simulink model "bh_4dof_LAGR_manipulator_CONTROL_DL_discrete"  (R2016b)
settings: Solver=ode23s  StartTime=0.0  StopTime=60  FixedStep=0.001  RelTol=1e-5  EnableMultiTasking=on
StopFcn:
  | bh_4dof_sim_post_process
values from neighbouring files (symbols this model uses):
  N = 3    [bh_4dof_sim_post_process.m]
undefined symbols (not defined in the file or in its folder): b1_damp, b2_damp, b3_damp, b4_damp, g, Hz, L1x, L1y, L1z, L2x, L2y, L2z, L3x, L3y, L3z, mass1, mass2, mass3, mass4, Rturn, theta1_0, theta1_dot_0, theta2_0, theta2_dot_0, theta3_0, theta3_dot_0, theta4_0, theta4_dot_0, X, Y, Z
libraries: simulink_extras x42, sm_lib x25, simulink x18, nesl_utility x17, discretizing x8
(part 4 of 4)

== system bh_4dof_LAGR_manipulator_CONTROL_DL_discrete/SIMULINK_MODEL/inside_MCKGQ/Subsystem1 ==
  M : Inport
  C : Inport  Port=2
  K : Inport  Port=3
  G : Inport  Port=4
  Q : Inport  Port=5
  T : Inport  Port=6
  Bus Selector : BusSelector  OutputSignals=theta_DOT_col
  Bus Selector1 : BusSelector  OutputSignals=theta_col
  Demux : Demux
  MATLAB Function : MATLAB Function  TreatAsAtomicUnit=on
  Product : Product  Multiplication=Matrix(*)
  Product1 : Product  Multiplication=Matrix(*)
  Product2 : Product  Inputs=/  Multiplication=Matrix(*)
  Product3 : Product  Multiplication=Matrix(*)
  SC_cond : Scope
  Sum : Sum  Inputs=+|+|+
  Sum1 : Sum  Inputs=|-+
  TH1_DD : Outport
  TH2_DD : Outport  Port=2
  TH3_DD : Outport  Port=3
  TH4_DD : Outport  Port=4
  wires:
  T/1 -> [T]
  C/1 -> Product/1
  [T] -> Bus Selector/1
  Bus Selector/1 -> Product/2  "<theta_DOT_col>"
  K/1 -> Product1/1
  [T] -> Bus Selector1/1
  Bus Selector1/1 -> Product1/2  "<theta_col>"
  Q/1 -> Sum1/2
  Product1/1 -> Sum/2
  G/1 -> Sum/3
  Product/1 -> Sum/1
  Sum/1 -> Sum1/1
  M/1 -> Product2/1, MATLAB Function/1(M)
  Product2/1 -> Product3/1
  Sum1/1 -> Product3/2
  Product3/1 -> Demux/1
  Demux/1 -> TH1_DD/1
  Demux/2 -> TH2_DD/1
  MATLAB Function/1(the_cond) -> SC_cond/1
  Demux/3 -> TH3_DD/1
  Demux/4 -> TH4_DD/1

== matlab function bh_4dof_LAGR_manipulator_CONTROL_DL_discrete/TRAJECTORY/THE_J ==
  data: L1Y_s input; the_J output; L2Y_s input; L3Y_s input; theta1 input; theta2 input; theta3 input; theta4 input
function the_J = THE_J(L1Y_s,L2Y_s,L3Y_s,theta1,theta2,theta3,theta4)
%#codegen

%    This function was generated by the Symbolic Math Toolbox version 7.0.
%    13-Sep-2016 14:49:06

the_J = reshape([sin(theta4).*(L2Y_s.*sin(theta1+theta2)+L1Y_s.*sin(theta1)+L3Y_s.*sin(theta1+theta2+theta3)),-cos(theta4).*(L2Y_s.*sin(theta1+theta2)+L1Y_s.*sin(theta1)+L3Y_s.*sin(theta1+theta2+theta3)),L2Y_s.*cos(theta1+theta2)+L1Y_s.*cos(theta1)+L3Y_s.*cos(theta1+theta2+theta3),sin(theta4).*(L2Y_s.*sin(theta1+theta2)+L3Y_s.*sin(theta1+theta2+theta3)),-cos(theta4).*(L2Y_s.*sin(theta1+theta2)+L3Y_s.*sin(theta1+theta2+theta3)),L2Y_s.*cos(theta1+theta2)+L3Y_s.*cos(theta1+theta2+theta3),L3Y_s.*sin(theta1+theta2+theta3).*sin(theta4),-L3Y_s.*sin(theta1+theta2+theta3).*cos(theta4),L3Y_s.*cos(theta1+theta2+theta3),-cos(theta4).*(L2Y_s.*cos(theta1+theta2)+L1Y_s.*cos(theta1)+L3Y_s.*cos(theta1+theta2+theta3)),-sin(theta4).*(L2Y_s.*cos(theta1+theta2)+L1Y_s.*cos(theta1)+L3Y_s.*cos(theta1+theta2+theta3)),0.0],[3,4]);

== matlab function bh_4dof_LAGR_manipulator_CONTROL_DL_discrete/Create_PLANT_BUS1/CALC_BUS/THE_A_EFF_and_O_and_G ==
  data: L1Y_s input; AF_pos_eff output; L2Y_s input; L3Y_s input; theta1 input; theta2 input; theta3 input; AF_pos_O1 output; AF_pos_O2 output; AF_pos_O3 output; AF_pos_G1 output; AF_pos_G2 output; AF_pos_G3 output
function [AF_pos_eff,AF_pos_O1,AF_pos_O2,AF_pos_O3,AF_pos_G1,AF_pos_G2,AF_pos_G3] = THE_A_EFF_and_O_and_G(L1Y_s,L2Y_s,L3Y_s,theta1,theta2,theta3)
%#codegen

%    This function was generated by the Symbolic Math Toolbox version 7.0.
%    15-Sep-2016 15:54:05

AF_pos_eff = [0.0;L2Y_s.*cos(theta1+theta2)+L1Y_s.*cos(theta1)+L3Y_s.*cos(theta1+theta2+theta3);L2Y_s.*sin(theta1+theta2)+L1Y_s.*sin(theta1)+L3Y_s.*sin(theta1+theta2+theta3)];
if nargout > 1
    AF_pos_O1 = [0.0;0.0;0.0];
end
if nargout > 2
    AF_pos_O2 = [0.0;L1Y_s.*cos(theta1);L1Y_s.*sin(theta1)];
end
if nargout > 3
    AF_pos_O3 = [0.0;L2Y_s.*cos(theta1+theta2)+L1Y_s.*cos(theta1);L2Y_s.*sin(theta1+theta2)+L1Y_s.*sin(theta1)];
end
if nargout > 4
    AF_pos_G1 = [0.0;L1Y_s.*cos(theta1).*(1.0./2.0);L1Y_s.*sin(theta1).*(1.0./2.0)];
end
if nargout > 5
    AF_pos_G2 = [0.0;L2Y_s.*cos(theta1+theta2).*(1.0./2.0)+L1Y_s.*cos(theta1);L2Y_s.*sin(theta1+theta2).*(1.0./2.0)+L1Y_s.*sin(theta1)];
end
if nargout > 6
    AF_pos_G3 = [0.0;L2Y_s.*cos(theta1+theta2)+L1Y_s.*cos(theta1)+L3Y_s.*cos(theta1+theta2+theta3).*(1.0./2.0);L2Y_s.*sin(theta1+theta2)+L1Y_s.*sin(theta1)+L3Y_s.*sin(theta1+theta2+theta3).*(1.0./2.0)];
end

== matlab function bh_4dof_LAGR_manipulator_CONTROL_DL_discrete/TRAJECTORY/CALC_THETA_DOT ==
  data: J input; TH_DOT output; XY_DOT input; lambda_sq input; alt_TH_DOT output
function [TH_DOT, alt_TH_DOT] = calc_TH_DOT(J, XY_DOT, lambda_sq)
%#codegen

    %% so our problem is this:
    %     J*q_dot = x_dot
    %
    % so a solution is:
    %
    %      q_dot = pinv(J) * x_dot
    
    TH_DOT = pinv(J) * XY_DOT;

    %% we can also penalise the q_dot by applying a weight to it.
    %  this will give us a solution where we get a "smaller" q_dot.  This
    %  acts as a "dampening" agent ... and we notice it most at startup.
    
    % consider solving the REGULARISED problem
    %     [       J_mxn  ] * q_dot =  [ x_dot ]
    %     [lamb^2*I_nxn  ]            [ 0_nx1 ]
    %
    % which we'll wite as:
    %
    %              new_A * q_dot = new_b
    %
    % so a solution is:
    %
    %      q_dot = pinv(new_A) * new_b
    
    [m, n]     = size(J); 
    I_mat      = eye( n ); 
    new_A      = [ J;
                   lambda_sq * I_mat];

    new_b      = [ XY_DOT;
                   zeros(n,1) ];

    alt_TH_DOT = pinv( new_A  ) * new_b;
end

== matlab function bh_4dof_LAGR_manipulator_CONTROL_DL_discrete/SIMULINK_MODEL/inside_MCKGQ/Subsystem1/MATLAB Function ==
  data: M input; the_cond output
function the_cond = COND(M)
%#codegen

the_cond = cond(M);

end

== matlab function bh_4dof_LAGR_manipulator_CONTROL_DL_discrete/Create_PLANT_BUS1/CALC_BUS/THE_W_EFF_and_O_and_G ==
  data: L1Y_s input; WF_pos_eff output; L2Y_s input; L3Y_s input; theta1 input; theta2 input; theta3 input; theta4 input; WF_pos_O1 output; WF_pos_O2 output; WF_pos_O3 output; WF_pos_G1 output; WF_pos_G2 output; WF_pos_G3 output
function [WF_pos_eff,WF_pos_O1,WF_pos_O2,WF_pos_O3,WF_pos_G1,WF_pos_G2,WF_pos_G3] = THE_W_EFF_and_O_and_G(L1Y_s,L2Y_s,L3Y_s,theta1,theta2,theta3,theta4)
%#codegen

%    This function was generated by the Symbolic Math Toolbox version 7.0.
%    15-Sep-2016 15:32:27

WF_pos_eff = [-sin(theta4).*(L2Y_s.*cos(theta1+theta2)+L1Y_s.*cos(theta1)+L3Y_s.*cos(theta1+theta2+theta3));cos(theta4).*(L2Y_s.*cos(theta1+theta2)+L1Y_s.*cos(theta1)+L3Y_s.*cos(theta1+theta2+theta3));L2Y_s.*sin(theta1+theta2)+L1Y_s.*sin(theta1)+L3Y_s.*sin(theta1+theta2+theta3)];
if nargout > 1
    WF_pos_O1 = [0.0;0.0;0.0];
end
if nargout > 2
    WF_pos_O2 = [-L1Y_s.*cos(theta1).*sin(theta4);L1Y_s.*cos(theta1).*cos(theta4);L1Y_s.*sin(theta1)];
end
if nargout > 3
    WF_pos_O3 = [-sin(theta4).*(L2Y_s.*cos(theta1+theta2)+L1Y_s.*cos(theta1));cos(theta4).*(L2Y_s.*cos(theta1+theta2)+L1Y_s.*cos(theta1));L2Y_s.*sin(theta1+theta2)+L1Y_s.*sin(theta1)];
end
if nargout > 4
    WF_pos_G1 = [L1Y_s.*cos(theta1).*sin(theta4).*(-1.0./2.0);L1Y_s.*cos(theta1).*cos(theta4).*(1.0./2.0);L1Y_s.*sin(theta1).*(1.0./2.0)];
end
if nargout > 5
    WF_pos_G2 = [-sin(theta4).*(L2Y_s.*cos(theta1+theta2).*(1.0./2.0)+L1Y_s.*cos(theta1));cos(theta4).*(L2Y_s.*cos(theta1+theta2).*(1.0./2.0)+L1Y_s.*cos(theta1));L2Y_s.*sin(theta1+theta2).*(1.0./2.0)+L1Y_s.*sin(theta1)];
end
if nargout > 6
    WF_pos_G3 = [-sin(theta4).*(L2Y_s.*cos(theta1+theta2)+L1Y_s.*cos(theta1)+L3Y_s.*cos(theta1+theta2+theta3).*(1.0./2.0));cos(theta4).*(L2Y_s.*cos(theta1+theta2)+L1Y_s.*cos(theta1)+L3Y_s.*cos(theta1+theta2+theta3).*(1.0./2.0));L2Y_s.*sin(theta1+theta2)+L1Y_s.*sin(theta1)+L3Y_s.*sin(theta1+theta2+theta3).*(1.0./2.0)];
end

== matlab function bh_4dof_LAGR_manipulator_CONTROL_DL_discrete/Create_PLANT_BUS1/Subsystem1/MATLAB Function ==
  data: r input size=[3 1]; TQ output; F input size=[3 1]
function TQ = CROSS(r,F)
%#codegen

TQ = cross(r,F);

== matlab function bh_4dof_LAGR_manipulator_CONTROL_DL_discrete/Create_PLANT_BUS1/Subsystem1/MATLAB Function1 ==
  data: r input size=[3 1]; TQ output; F input size=[3 1]
function TQ = CROSS(r,F)
%#codegen

TQ = cross(r,F);

== matlab function bh_4dof_LAGR_manipulator_CONTROL_DL_discrete/Create_PLANT_BUS1/Subsystem1/MATLAB Function2 ==
  data: r input size=[3 1]; TQ output; F input size=[3 1]
function TQ = CROSS(r,F)
%#codegen

TQ = cross(r,F);

== matlab function bh_4dof_LAGR_manipulator_CONTROL_DL_discrete/Create_PLANT_BUS1/Subsystem1/MATLAB Function3 ==
  data: r input size=[3 1]; TQ output; F input size=[3 1]
function TQ = CROSS(r,F)
%#codegen

TQ = cross(r,F);

== matlab function bh_4dof_LAGR_manipulator_CONTROL_DL_discrete/Create_PLANT_BUS1/Subsystem1/MATLAB Function4 ==
  data: r input size=[3 1]; TQ output; F input size=[3 1]
function TQ = CROSS(r,F)
%#codegen

TQ = cross(r,F);

== matlab function bh_4dof_LAGR_manipulator_CONTROL_DL_discrete/Create_PLANT_BUS1/Subsystem1/MATLAB Function5 ==
  data: r input size=[3 1]; TQ output; F input size=[3 1]
function TQ = CROSS(r,F)
%#codegen

TQ = cross(r,F);

== matlab function bh_4dof_LAGR_manipulator_CONTROL_DL_discrete/TRAJECTORY/THE_XEYE ==
  data: L1Y_s input; XE output; L2Y_s input; L3Y_s input; theta1 input; theta2 input; theta3 input; theta4 input; YE output; ZE output
function [XE,YE,ZE] = THE_XEYE(L1Y_s,L2Y_s,L3Y_s,theta1,theta2,theta3,theta4)
%#codegen

%    This function was generated by the Symbolic Math Toolbox version 7.0.
%    13-Sep-2016 15:29:58

XE = -sin(theta4).*(L2Y_s.*cos(theta1+theta2)+L1Y_s.*cos(theta1)+L3Y_s.*cos(theta1+theta2+theta3));
if nargout > 1
    YE = cos(theta4).*(L2Y_s.*cos(theta1+theta2)+L1Y_s.*cos(theta1)+L3Y_s.*cos(theta1+theta2+theta3));
end
if nargout > 2
    ZE = L2Y_s.*sin(theta1+theta2)+L1Y_s.*sin(theta1)+L3Y_s.*sin(theta1+theta2+theta3);
end

== matlab function bh_4dof_LAGR_manipulator_CONTROL_DL_discrete/Create_PLANT_BUS/CALC_BUS/THE_A_EFF_and_O_and_G ==
  data: L1Y_s input; AF_pos_eff output; L2Y_s input; L3Y_s input; theta1 input; theta2 input; theta3 input; AF_pos_O1 output; AF_pos_O2 output; AF_pos_O3 output; AF_pos_G1 output; AF_pos_G2 output; AF_pos_G3 output
function [AF_pos_eff,AF_pos_O1,AF_pos_O2,AF_pos_O3,AF_pos_G1,AF_pos_G2,AF_pos_G3] = THE_A_EFF_and_O_and_G(L1Y_s,L2Y_s,L3Y_s,theta1,theta2,theta3)
%#codegen

%    This function was generated by the Symbolic Math Toolbox version 7.0.
%    15-Sep-2016 15:54:05

AF_pos_eff = [0.0;L2Y_s.*cos(theta1+theta2)+L1Y_s.*cos(theta1)+L3Y_s.*cos(theta1+theta2+theta3);L2Y_s.*sin(theta1+theta2)+L1Y_s.*sin(theta1)+L3Y_s.*sin(theta1+theta2+theta3)];
if nargout > 1
    AF_pos_O1 = [0.0;0.0;0.0];
end
if nargout > 2
    AF_pos_O2 = [0.0;L1Y_s.*cos(theta1);L1Y_s.*sin(theta1)];
end
if nargout > 3
    AF_pos_O3 = [0.0;L2Y_s.*cos(theta1+theta2)+L1Y_s.*cos(theta1);L2Y_s.*sin(theta1+theta2)+L1Y_s.*sin(theta1)];
end
if nargout > 4
    AF_pos_G1 = [0.0;L1Y_s.*cos(theta1).*(1.0./2.0);L1Y_s.*sin(theta1).*(1.0./2.0)];
end
if nargout > 5
    AF_pos_G2 = [0.0;L2Y_s.*cos(theta1+theta2).*(1.0./2.0)+L1Y_s.*cos(theta1);L2Y_s.*sin(theta1+theta2).*(1.0./2.0)+L1Y_s.*sin(theta1)];
end
if nargout > 6
    AF_pos_G3 = [0.0;L2Y_s.*cos(theta1+theta2)+L1Y_s.*cos(theta1)+L3Y_s.*cos(theta1+theta2+theta3).*(1.0./2.0);L2Y_s.*sin(theta1+theta2)+L1Y_s.*sin(theta1)+L3Y_s.*sin(theta1+theta2+theta3).*(1.0./2.0)];
end

== matlab function bh_4dof_LAGR_manipulator_CONTROL_DL_discrete/Create_PLANT_BUS/CALC_BUS/THE_W_EFF_and_O_and_G ==
  data: L1Y_s input; WF_pos_eff output; L2Y_s input; L3Y_s input; theta1 input; theta2 input; theta3 input; theta4 input; WF_pos_O1 output; WF_pos_O2 output; WF_pos_O3 output; WF_pos_G1 output; WF_pos_G2 output; WF_pos_G3 output
function [WF_pos_eff,WF_pos_O1,WF_pos_O2,WF_pos_O3,WF_pos_G1,WF_pos_G2,WF_pos_G3] = THE_W_EFF_and_O_and_G(L1Y_s,L2Y_s,L3Y_s,theta1,theta2,theta3,theta4)
%#codegen

%    This function was generated by the Symbolic Math Toolbox version 7.0.
%    15-Sep-2016 15:32:27

WF_pos_eff = [-sin(theta4).*(L2Y_s.*cos(theta1+theta2)+L1Y_s.*cos(theta1)+L3Y_s.*cos(theta1+theta2+theta3));cos(theta4).*(L2Y_s.*cos(theta1+theta2)+L1Y_s.*cos(theta1)+L3Y_s.*cos(theta1+theta2+theta3));L2Y_s.*sin(theta1+theta2)+L1Y_s.*sin(theta1)+L3Y_s.*sin(theta1+theta2+theta3)];
if nargout > 1
    WF_pos_O1 = [0.0;0.0;0.0];
end
if nargout > 2
    WF_pos_O2 = [-L1Y_s.*cos(theta1).*sin(theta4);L1Y_s.*cos(theta1).*cos(theta4);L1Y_s.*sin(theta1)];
end
if nargout > 3
    WF_pos_O3 = [-sin(theta4).*(L2Y_s.*cos(theta1+theta2)+L1Y_s.*cos(theta1));cos(theta4).*(L2Y_s.*cos(theta1+theta2)+L1Y_s.*cos(theta1));L2Y_s.*sin(theta1+theta2)+L1Y_s.*sin(theta1)];
end
if nargout > 4
    WF_pos_G1 = [L1Y_s.*cos(theta1).*sin(theta4).*(-1.0./2.0);L1Y_s.*cos(theta1).*cos(theta4).*(1.0./2.0);L1Y_s.*sin(theta1).*(1.0./2.0)];
end
if nargout > 5
    WF_pos_G2 = [-sin(theta4).*(L2Y_s.*cos(theta1+theta2).*(1.0./2.0)+L1Y_s.*cos(theta1));cos(theta4).*(L2Y_s.*cos(theta1+theta2).*(1.0./2.0)+L1Y_s.*cos(theta1));L2Y_s.*sin(theta1+theta2).*(1.0./2.0)+L1Y_s.*sin(theta1)];
end
if nargout > 6
    WF_pos_G3 = [-sin(theta4).*(L2Y_s.*cos(theta1+theta2)+L1Y_s.*cos(theta1)+L3Y_s.*cos(theta1+theta2+theta3).*(1.0./2.0));cos(theta4).*(L2Y_s.*cos(theta1+theta2)+L1Y_s.*cos(theta1)+L3Y_s.*cos(theta1+theta2+theta3).*(1.0./2.0));L2Y_s.*sin(theta1+theta2)+L1Y_s.*sin(theta1)+L3Y_s.*sin(theta1+theta2+theta3).*(1.0./2.0)];
end

== matlab function bh_4dof_LAGR_manipulator_CONTROL_DL_discrete/Create_PLANT_BUS/Subsystem1/MATLAB Function ==
  data: r input size=[3 1]; TQ output; F input size=[3 1]
function TQ = CROSS(r,F)
%#codegen

TQ = cross(r,F);

== matlab function bh_4dof_LAGR_manipulator_CONTROL_DL_discrete/Create_PLANT_BUS/Subsystem1/MATLAB Function1 ==
  data: r input size=[3 1]; TQ output; F input size=[3 1]
function TQ = CROSS(r,F)
%#codegen

TQ = cross(r,F);

== matlab function bh_4dof_LAGR_manipulator_CONTROL_DL_discrete/Create_PLANT_BUS/Subsystem1/MATLAB Function2 ==
  data: r input size=[3 1]; TQ output; F input size=[3 1]
function TQ = CROSS(r,F)
%#codegen

TQ = cross(r,F);

== matlab function bh_4dof_LAGR_manipulator_CONTROL_DL_discrete/Create_PLANT_BUS/Subsystem1/MATLAB Function3 ==
  data: r input size=[3 1]; TQ output; F input size=[3 1]
function TQ = CROSS(r,F)
%#codegen

TQ = cross(r,F);

== matlab function bh_4dof_LAGR_manipulator_CONTROL_DL_discrete/Create_PLANT_BUS/Subsystem1/MATLAB Function4 ==
  data: r input size=[3 1]; TQ output; F input size=[3 1]
function TQ = CROSS(r,F)
%#codegen

TQ = cross(r,F);

== matlab function bh_4dof_LAGR_manipulator_CONTROL_DL_discrete/Create_PLANT_BUS/Subsystem1/MATLAB Function5 ==
  data: r input size=[3 1]; TQ output; F input size=[3 1]
function TQ = CROSS(r,F)
%#codegen

TQ = cross(r,F);

== matlab function bh_4dof_LAGR_manipulator_CONTROL_DL_discrete/SIMULINK_MODEL/inside_MCKGQ/MCKGQ ==
  data: L1X_s input; M output; L2X_s input; L3X_s input; L1Y_s input; L2Y_s input; L3Y_s input; L1Z_s input; L2Z_s input; L3Z_s input; R4_s input; TH1_s input; TH2_s input; TH3_s input; TH1_s_D input; TH2_s_D input; TH3_s_D input; TH4_s_D input; b1_s input; b2_s input; b3_s input; b4_s input; g_s input; m1_s input; m2_s input; m3_s input; m4_s input; taum1_s input; taum2_s input; taum3_s input; taum4_s input; C output; K output; G output; Q output
function [M,C,K,G,Q] = MCKGQ(L1X_s,L2X_s,L3X_s,L1Y_s,L2Y_s,L3Y_s,L1Z_s,L2Z_s,L3Z_s,R4_s,TH1_s,TH2_s,TH3_s,TH1_s_D,TH2_s_D,TH3_s_D,TH4_s_D,b1_s,b2_s,b3_s,b4_s,g_s,m1_s,m2_s,m3_s,m4_s,taum1_s,taum2_s,taum3_s,taum4_s)
%#codegen

%    This function was generated by the Symbolic Math Toolbox version 7.1.
%    31-Jan-2017 14:34:44

M = reshape([L1Y_s.^2.*m1_s.*(1.0./3.0)+L1Y_s.^2.*m2_s+L1Y_s.^2.*m3_s+L2Y_s.^2.*m2_s.*(1.0./3.0)+L2Y_s.^2.*m3_s+L3Y_s.^2.*m3_s.*(1.0./3.0)+L1Z_s.^2.*m1_s.*(1.0./1.2e1)+L2Z_s.^2.*m2_s.*(1.0./1.2e1)+L3Z_s.^2.*m3_s.*(1.0./1.2e1)+L1Y_s.*L2Y_s.*m2_s.*cos(TH2_s)+L1Y_s.*L2Y_s.*m3_s.*cos(TH2_s).*2.0+L2Y_s.*L3Y_s.*m3_s.*cos(TH3_s)+L1Y_s.*L3Y_s.*m3_s.*cos(TH2_s+TH3_s),L2Y_s.^2.*m2_s.*(1.0./3.0)+L2Y_s.^2.*m3_s+L3Y_s.^2.*m3_s.*(1.0./3.0)+L2Z_s.^2.*m2_s.*(1.0./1.2e1)+L3Z_s.^2.*m3_s.*(1.0./1.2e1)+L1Y_s.*L2Y_s.*m2_s.*cos(TH2_s).*(1.0./2.0)+L1Y_s.*L2Y_s.*m3_s.*cos(TH2_s)+L2Y_s.*L3Y_s.*m3_s.*cos(TH3_s)+L1Y_s.*L3Y_s.*m3_s.*cos(TH2_s+TH3_s).*(1.0./2.0),m3_s.*(L3Y_s.^2.*4.0+L3Z_s.^2+L1Y_s.*L3Y_s.*cos(TH2_s+TH3_s).*6.0+L2Y_s.*L3Y_s.*cos(TH3_s).*6.0).*(1.0./1.2e1),0.0,L2Y_s.^2.*m2_s.*(1.0./3.0)+L2Y_s.^2.*m3_s+L3Y_s.^2.*m3_s.*(1.0./3.0)+L2Z_s.^2.*m2_s.*(1.0./1.2e1)+L3Z_s.^2.*m3_s.*(1.0./1.2e1)+L1Y_s.*L2Y_s.*m2_s.*cos(TH2_s).*(1.0./2.0)+L1Y_s.*L2Y_s.*m3_s.*cos(TH2_s)+L2Y_s.*L3Y_s.*m3_s.*cos(TH3_s)+L1Y_s.*L3Y_s.*m3_s.*cos(TH2_s+TH3_s).*(1.0./2.0),L2Y_s.^2.*m2_s.*(1.0./3.0)+L2Y_s.^2.*m3_s+L3Y_s.^2.*m3_s.*(1.0./3.0)+L2Z_s.^2.*m2_s.*(1.0./1.2e1)+L3Z_s.^2.*m3_s.*(1.0./1.2e1)+L2Y_s.*L3Y_s.*m3_s.*cos(TH3_s),m3_s.*(L3Y_s.^2.*4.0+L3Z_s.^2+L2Y_s.*L3Y_s.*cos(TH3_s).*6.0).*(1.0./1.2e1),0.0,m3_s.*(L3Y_s.^2.*4.0+L3Z_s.^2+L1Y_s.*L3Y_s.*cos(TH2_s+TH3_s).*6.0+L2Y_s.*L3Y_s.*cos(TH3_s).*6.0).*(1.0./1.2e1),m3_s.*(L3Y_s.^2.*4.0+L3Z_s.^2+L2Y_s.*L3Y_s.*cos(TH3_s).*6.0).*(1.0./1.2e1),m3_s.*(L3Y_s.^2.*4.0+L3Z_s.^2).*(1.0./1.2e1),0.0,0.0,0.0,0.0,L1X_s.^2.*m1_s.*(1.0./1.2e1)+L2X_s.^2.*m2_s.*(1.0./1.2e1)+L3X_s.^2.*m3_s.*(1.0./1.2e1)+L1Y_s.^2.*m1_s.*(1.0./6.0)+L1Y_s.^2.*m2_s.*(1.0./2.0)+L1Y_s.^2.*m3_s.*(1.0./2.0)+L2Y_s.^2.*m2_s.*(1.0./6.0)+L2Y_s.^2.*m3_s.*(1.0./2.0)+L3Y_s.^2.*m3_s.*(1.0./6.0)+L1Z_s.^2.*m1_s.*(1.0./2.4e1)+L2Z_s.^2.*m2_s.*(1.0./2.4e1)+L3Z_s.^2.*m3_s.*(1.0./2.4e1)+R4_s.^2.*m4_s.*(1.0./2.0)+L3Y_s.^2.*m3_s.*cos(TH1_s.*2.0+TH2_s.*2.0+TH3_s.*2.0).*(1.0./6.0)-L3Z_s.^2.*m3_s.*cos(TH1_s.*2.0+TH2_s.*2.0+TH3_s.*2.0).*(1.0./2.4e1)+L1Y_s.^2.*m1_s.*cos(TH1_s.*2.0).*(1.0./6.0)+L1Y_s.^2.*m2_s.*cos(TH1_s.*2.0).*(1.0./2.0)+L1Y_s.^2.*m3_s.*cos(TH1_s.*2.0).*(1.0./2.0)-L1Z_s.^2.*m1_s.*cos(TH1_s.*2.0).*(1.0./2.4e1)+L2Y_s.^2.*m2_s.*cos(TH1_s.*2.0+TH2_s.*2.0).*(1.0./6.0)+L2Y_s.^2.*m3_s.*cos(TH1_s.*2.0+TH2_s.*2.0).*(1.0./2.0)-L2Z_s.^2.*m2_s.*cos(TH1_s.*2.0+TH2_s.*2.0).*(1.0./2.4e1)+L1Y_s.*L2Y_s.*m2_s.*cos(TH2_s).*(1.0./2.0)+L1Y_s.*L2Y_s.*m3_s.*cos(TH2_s)+L2Y_s.*L3Y_s.*m3_s.*cos(TH3_s).*(1.0./2.0)+L1Y_s.*L2Y_s.*m2_s.*cos(TH1_s.*2.0+TH2_s).*(1.0./2.0)+L1Y_s.*L2Y_s.*m3_s.*cos(TH1_s.*2.0+TH2_s)+L1Y_s.*L3Y_s.*m3_s.*cos(TH1_s.*2.0+TH2_s+TH3_s).*(1.0./2.0)+L1Y_s.*L3Y_s.*m3_s.*cos(TH2_s+TH3_s).*(1.0./2.0)+L2Y_s.*L3Y_s.*m3_s.*cos(TH1_s.*2.0+TH2_s.*2.0+TH3_s).*(1.0./2.0)],[4,4]);
if nargout > 1
    C = reshape([-L1Y_s.*L3Y_s.*TH2_s_D.*m3_s.*sin(TH2_s+TH3_s)-L1Y_s.*L3Y_s.*TH3_s_D.*m3_s.*sin(TH2_s+TH3_s)-L1Y_s.*L2Y_s.*TH2_s_D.*m2_s.*sin(TH2_s)-L1Y_s.*L2Y_s.*TH2_s_D.*m3_s.*sin(TH2_s).*2.0-L2Y_s.*L3Y_s.*TH3_s_D.*m3_s.*sin(TH3_s),L1Y_s.*L3Y_s.*TH1_s_D.*m3_s.*sin(TH2_s+TH3_s).*(1.0./2.0)+L1Y_s.*L2Y_s.*TH1_s_D.*m2_s.*sin(TH2_s).*(1.0./2.0)+L1Y_s.*L2Y_s.*TH1_s_D.*m3_s.*sin(TH2_s)-L2Y_s.*L3Y_s.*TH3_s_D.*m3_s.*sin(TH3_s),L3Y_s.*m3_s.*(L1Y_s.*TH1_s_D.*sin(TH2_s+TH3_s)+L2Y_s.*TH1_s_D.*sin(TH3_s)+L2Y_s.*TH2_s_D.*sin(TH3_s).*2.0).*(1.0./2.0),TH4_s_D.*(L3Y_s.^2.*m3_s.*sin(TH1_s.*2.0+TH2_s.*2.0+TH3_s.*2.0).*4.0-L3Z_s.^2.*m3_s.*sin(TH1_s.*2.0+TH2_s.*2.0+TH3_s.*2.0)+L1Y_s.^2.*m1_s.*sin(TH1_s.*2.0).*4.0+L1Y_s.^2.*m2_s.*sin(TH1_s.*2.0).*1.2e1+L1Y_s.^2.*m3_s.*sin(TH1_s.*2.0).*1.2e1-L1Z_s.^2.*m1_s.*sin(TH1_s.*2.0)+L2Y_s.^2.*m2_s.*sin(TH1_s.*2.0+TH2_s.*2.0).*4.0+L2Y_s.^2.*m3_s.*sin(TH1_s.*2.0+TH2_s.*2.0).*1.2e1-L2Z_s.^2.*m2_s.*sin(TH1_s.*2.0+TH2_s.*2.0)+L1Y_s.*L2Y_s.*m2_s.*sin(TH1_s.*2.0+TH2_s).*1.2e1+L1Y_s.*L2Y_s.*m3_s.*sin(TH1_s.*2.0+TH2_s).*2.4e1+L1Y_s.*L3Y_s.*m3_s.*sin(TH1_s.*2.0+TH2_s+TH3_s).*1.2e1+L2Y_s.*L3Y_s.*m3_s.*sin(TH1_s.*2.0+TH2_s.*2.0+TH3_s).*1.2e1).*(-1.0./1.2e1),L1Y_s.*L3Y_s.*TH2_s_D.*m3_s.*sin(TH2_s+TH3_s).*(-1.0./2.0)-L1Y_s.*L3Y_s.*TH3_s_D.*m3_s.*sin(TH2_s+TH3_s)-L1Y_s.*L2Y_s.*TH2_s_D.*m2_s.*sin(TH2_s).*(1.0./2.0)-L1Y_s.*L2Y_s.*TH2_s_D.*m3_s.*sin(TH2_s)-L2Y_s.*L3Y_s.*TH3_s_D.*m3_s.*sin(TH3_s),-L2Y_s.*L3Y_s.*TH3_s_D.*m3_s.*sin(TH3_s),L2Y_s.*L3Y_s.*TH2_s_D.*m3_s.*sin(TH3_s).*(1.0./2.0),TH4_s_D.*(L3Y_s.^2.*m3_s.*sin(TH1_s.*2.0+TH2_s.*2.0+TH3_s.*2.0).*4.0-L3Z_s.^2.*m3_s.*sin(TH1_s.*2.0+TH2_s.*2.0+TH3_s.*2.0)+L2Y_s.^2.*m2_s.*sin(TH1_s.*2.0+TH2_s.*2.0).*4.0+L2Y_s.^2.*m3_s.*sin(TH1_s.*2.0+TH2_s.*2.0).*1.2e1-L2Z_s.^2.*m2_s.*sin(TH1_s.*2.0+TH2_s.*2.0)+L1Y_s.*L2Y_s.*m2_s.*sin(TH2_s).*6.0+L1Y_s.*L2Y_s.*m3_s.*sin(TH2_s).*1.2e1+L1Y_s.*L2Y_s.*m2_s.*sin(TH1_s.*2.0+TH2_s).*6.0+L1Y_s.*L2Y_s.*m3_s.*sin(TH1_s.*2.0+TH2_s).*1.2e1+L1Y_s.*L3Y_s.*m3_s.*sin(TH1_s.*2.0+TH2_s+TH3_s).*6.0+L1Y_s.*L3Y_s.*m3_s.*sin(TH2_s+TH3_s).*6.0+L2Y_s.*L3Y_s.*m3_s.*sin(TH1_s.*2.0+TH2_s.*2.0+TH3_s).*1.2e1).*(-1.0./1.2e1),L3Y_s.*TH3_s_D.*m3_s.*(L1Y_s.*sin(TH2_s+TH3_s)+L2Y_s.*sin(TH3_s)).*(-1.0./2.0),L2Y_s.*L3Y_s.*TH3_s_D.*m3_s.*sin(TH3_s).*(-1.0./2.0),0.0,TH4_s_D.*m3_s.*(L3Y_s.^2.*sin(TH1_s.*2.0+TH2_s.*2.0+TH3_s.*2.0).*4.0-L3Z_s.^2.*sin(TH1_s.*2.0+TH2_s.*2.0+TH3_s.*2.0)+L1Y_s.*L3Y_s.*sin(TH1_s.*2.0+TH2_s+TH3_s).*6.0+L1Y_s.*L3Y_s.*sin(TH2_s+TH3_s).*6.0+L2Y_s.*L3Y_s.*sin(TH1_s.*2.0+TH2_s.*2.0+TH3_s).*6.0+L2Y_s.*L3Y_s.*sin(TH3_s).*6.0).*(-1.0./1.2e1),TH4_s_D.*(L3Y_s.^2.*m3_s.*sin(TH1_s.*2.0+TH2_s.*2.0+TH3_s.*2.0).*4.0-L3Z_s.^2.*m3_s.*sin(TH1_s.*2.0+TH2_s.*2.0+TH3_s.*2.0)+L1Y_s.^2.*m1_s.*sin(TH1_s.*2.0).*4.0+L1Y_s.^2.*m2_s.*sin(TH1_s.*2.0).*1.2e1+L1Y_s.^2.*m3_s.*sin(TH1_s.*2.0).*1.2e1-L1Z_s.^2.*m1_s.*sin(TH1_s.*2.0)+L2Y_s.^2.*m2_s.*sin(TH1_s.*2.0+TH2_s.*2.0).*4.0+L2Y_s.^2.*m3_s.*sin(TH1_s.*2.0+TH2_s.*2.0).*1.2e1-L2Z_s.^2.*m2_s.*sin(TH1_s.*2.0+TH2_s.*2.0)+L1Y_s.*L2Y_s.*m2_s.*sin(TH1_s.*2.0+TH2_s).*1.2e1+L1Y_s.*L2Y_s.*m3_s.*sin(TH1_s.*2.0+TH2_s).*2.4e1+L1Y_s.*L3Y_s.*m3_s.*sin(TH1_s.*2.0+TH2_s+TH3_s).*1.2e1+L2Y_s.*L3Y_s.*m3_s.*sin(TH1_s.*2.0+TH2_s.*2.0+TH3_s).*1.2e1).*(1.0./2.4e1),TH4_s_D.*(L3Y_s.^2.*m3_s.*sin(TH1_s.*2.0+TH2_s.*2.0+TH3_s.*2.0).*4.0-L3Z_s.^2.*m3_s.*sin(TH1_s.*2.0+TH2_s.*2.0+TH3_s.*2.0)+L2Y_s.^2.*m2_s.*sin(TH1_s.*2.0+TH2_s.*2.0).*4.0+L2Y_s.^2.*m3_s.*sin(TH1_s.*2.0+TH2_s.*2.0).*1.2e1-L2Z_s.^2.*m2_s.*sin(TH1_s.*2.0+TH2_s.*2.0)+L1Y_s.*L2Y_s.*m2_s.*sin(TH2_s).*6.0+L1Y_s.*L2Y_s.*m3_s.*sin(TH2_s).*1.2e1+L1Y_s.*L2Y_s.*m2_s.*sin(TH1_s.*2.0+TH2_s).*6.0+L1Y_s.*L2Y_s.*m3_s.*sin(TH1_s.*2.0+TH2_s).*1.2e1+L1Y_s.*L3Y_s.*m3_s.*sin(TH1_s.*2.0+TH2_s+TH3_s).*6.0+L1Y_s.*L3Y_s.*m3_s.*sin(TH2_s+TH3_s).*6.0+L2Y_s.*L3Y_s.*m3_s.*sin(TH1_s.*2.0+TH2_s.*2.0+TH3_s).*1.2e1).*(1.0./2.4e1),TH4_s_D.*m3_s.*(L3Y_s.^2.*sin(TH1_s.*2.0+TH2_s.*2.0+TH3_s.*2.0).*4.0-L3Z_s.^2.*sin(TH1_s.*2.0+TH2_s.*2.0+TH3_s.*2.0)+L1Y_s.*L3Y_s.*sin(TH1_s.*2.0+TH2_s+TH3_s).*6.0+L1Y_s.*L3Y_s.*sin(TH2_s+TH3_s).*6.0+L2Y_s.*L3Y_s.*sin(TH1_s.*2.0+TH2_s.*2.0+TH3_s).*6.0+L2Y_s.*L3Y_s.*sin(TH3_s).*6.0).*(1.0./2.4e1),0.0],[4,4]);
end
if nargout > 2
    K = reshape([0.0,0.0,0.0,0.0,0.0,0.0,0.0,0.0,0.0,0.0,0.0,0.0,0.0,0.0,0.0,0.0],[4,4]);
end
if nargout > 3
    G = [g_s.*(L2Y_s.*m2_s.*cos(TH1_s+TH2_s)+L2Y_s.*m3_s.*cos(TH1_s+TH2_s).*2.0+L1Y_s.*m1_s.*cos(TH1_s)+L1Y_s.*m2_s.*cos(TH1_s).*2.0+L1Y_s.*m3_s.*cos(TH1_s).*2.0+L3Y_s.*m3_s.*cos(TH1_s+TH2_s+TH3_s)).*(1.0./2.0);L3Y_s.*g_s.*m3_s.*cos(TH1_s+TH2_s+TH3_s).*(1.0./2.0)+L2Y_s.*g_s.*m2_s.*cos(TH1_s+TH2_s).*(1.0./2.0)+L2Y_s.*g_s.*m3_s.*cos(TH1_s+TH2_s);L3Y_s.*g_s.*m3_s.*cos(TH1_s+TH2_s+TH3_s).*(1.0./2.0);0.0];
end
if nargout > 4
    Q = [taum1_s-TH1_s_D.*b1_s;taum2_s-TH2_s_D.*b2_s;taum3_s-TH3_s_D.*b3_s;taum4_s-TH4_s_D.*b4_s];
end
